simulink model "cardio"  (Simulink 7.2)
settings: Solver=ode45  StartTime=0.0  StopTime=10.0  RelTol=1e-3
undefined symbols (not defined in the file): ln
(part 1 of 2)
settings Model: Creator=hp  LastModifiedBy=hp

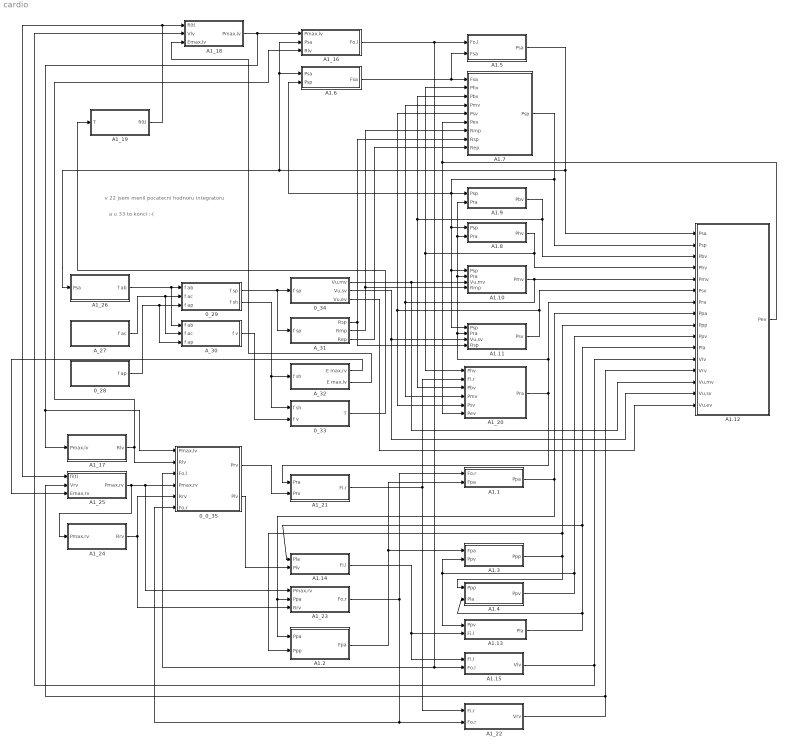
== system cardio ==
  note: v 22 jsem menil pocatecni hodnoru integratoru
  note: a u 33 to konci :-(
  0_0_35 : Subsystem
  0_28 : Subsystem
  0_29 : Subsystem
  0_33 : Subsystem
  0_34 : Subsystem
  A1.1 : Subsystem
  A1.10 : Subsystem
  A1.11 : Subsystem
  A1.12 : Subsystem
  A1.13 : Subsystem
  A1.14 : Subsystem
  A1.15 : Subsystem
  A1.2 : Subsystem
  A1.3 : Subsystem
  A1.4 : Subsystem
  A1.5 : Subsystem
  A1.6 : Subsystem
  A1.7 : Subsystem
  A1.8 : Subsystem
  A1.9 : Subsystem
  A1_16 : Subsystem
  A1_17 : Subsystem
  A1_18 : Subsystem
  A1_19 : Subsystem
  A1_20 : Subsystem
  A1_21 : Subsystem
  A1_22 : Subsystem
  A1_23 : Subsystem
  A1_24 : Subsystem
  A1_25 : Subsystem
  A1_26 : Subsystem
  A_27 : Subsystem
  A_30 : Subsystem
  A_31 : Subsystem
  A_32 : Subsystem
  wires:
  A1.10/1(Pmv) -> A1.12/5(Pmv), A1.7/4(Pmv), A1_20/4(Pmv)
  A1.11/1(Psv) -> A1.12/6(Psv), A1.7/5(Psv), A1_20/5(Psv)
  A1.3/1(Ppp) -> A1.4/1(Ppp), A1.12/9(Ppp), A1.2/2(Ppp)
  A1.15/1(Vlv) -> A1.12/12(Vlv), A1_18/2(Vlv)
  A1_26/1(f ab) -> 0_29/1(f ab), A_30/1(f ab)
  A_27/1(f ac) -> 0_29/2(f ac), A_30/2(f ac)
  0_28/1(f ap) -> 0_29/3(f ap), A_30/3(f ap)
  0_29/1(f sp) -> 0_34/1(f sp), A_31/1(f sp)
  0_29/2(f sh) -> A_32/1(f sh), 0_33/1(f sh)
  A1.4/1(Ppv) -> A1.12/10(Ppv), A1.3/2(Ppv), A1.13/1(Ppv)
  A1.13/1(Pla) -> A1.4/2(Pla), A1.12/11(Pla), A1.14/1(Pla)
  A1.8/1(Phv) -> A1.12/4(Phv), A1_20/1(Phv), A1.7/2(Phv)
  A1.9/1(Pbv) -> A1.12/3(Pbv), A1.7/3(Pbv), A1_20/3(Pbv)
  A1.7/1(Psp) -> A1.12/2(Psp), A1.9/1(Psp), A1.8/1(Psp), A1.10/1(Psp), A1.11/1(Psp), A1.6/2(Psp)
  A1.5/1(Psa) -> A1.12/1(Psa), A1.6/1(Psa), A1_16/2(Psa), A1_26/1(Psa)
  A1_20/1(Pra) -> A1.12/7(Pra), A1.10/2(Pra), A1.8/2(Pra), A1.9/2(Pra), A1.11/2(Pra), A1_21/1(Pra)
  A1.1/1(Ppa) -> A1.12/8(Ppa), A1.2/1(Ppa), A1_23/2(Ppa)
  A1_22/1(Vrv) -> A1.12/13(Vrv), A1_25/2(Vrv)
  A1_16/1(Fo,l) -> A1.5/1(Fo,l), A1.15/2(Fo,l), 0_0_35/3(Fo,l)
  A1.6/1(Fsa) -> A1.7/1(Fsa), A1.5/2(Fsa)
  A1.12/1(Pev) -> A1.7/6(Pev), A1_20/6(Pev)
  0_34/1(Vu,mv) -> A1.10/3(Vu,mv), A1.12/14(Vu,mv)
  0_34/2(Vu,sv) -> A1.11/3(Vu,sv), A1.12/15(Vu,sv)
  A1_21/1(Fi,r) -> A1_20/2(Fi,r), A1_22/1(Fi,r)
  A1.14/1(Fi,l) -> A1.15/1(Fi,l), A1.13/2(Fi,l)
  A1_23/1(Fo,r) -> A1.1/1(Fo,r), A1_22/2(Fo,r), 0_0_35/6(Fo,r)
  A1.2/1(Fpa) -> A1.3/1(Fpa), A1.1/2(Fpa)
  A1_18/1(Pmax,lv) -> A1_16/1(Pmax,lv), A1_17/1(Pmax,lv), 0_0_35/1(Pmax,lv)
  0_0_35/1(Prv) -> A1_21/2(Prv)
  0_0_35/2(Plv) -> A1.14/2(Plv)
  A1_25/1(Pmax,rv) -> A1_24/1(Pmax,rv), 0_0_35/4(Pmax,rv), A1_23/1(Pmax,rv)
  A1_24/1(Rrv) -> 0_0_35/5(Rrv), A1_23/3(Rrv)
  A1_17/1(Rlv) -> 0_0_35/2(Rlv), A1_16/3(Rlv)
  A1_19/1(fi(t)) -> A1_18/1(fi(t)), A1_25/1(fi(t))
  0_33/1(T) -> A1_19/1(T)
  A_31/1(Rsp) -> A1.7/8(Rsp), A1.11/4(Rsp)
  A_31/2(Rmp) -> A1.7/7(Rmp), A1.10/4(Rmp)
  A_31/3(Rep) -> A1.7/9(Rep)
  A_32/2(E max,lv) -> A1_18/3(Emax,lv)
  A_32/1(E max,rv) -> A1_25/3(Emax,rv)
  0_34/3(Vu,ev) -> A1.12/16(Vu,ev)
  A_30/1(f v) -> 0_33/2(f v)

== system cardio/0_0_35 ==
  Pmax,lv : Inport  OutDataType=fixdt(1, 16)  OutScaling=2^0
  Rlv : Inport  Port=2  OutDataType=fixdt(1, 16)  OutScaling=2^0
  Fo,l : Inport  Port=3  OutDataType=fixdt(1, 16)  OutScaling=2^0
  Pmax,rv : Inport  Port=4  OutDataType=fixdt(1, 16)  OutScaling=2^0
  Rrv : Inport  Port=5  OutDataType=fixdt(1, 16)  OutScaling=2^0
  Fo,r : Inport  Port=6  OutDataType=fixdt(1, 16)  OutScaling=2^0
  Add : Sum  Inputs=+-  OutDataType=fixdt(1, 16)  OutScaling=2^-10
  Add1 : Sum  Inputs=+-  OutDataType=fixdt(1, 16)  OutScaling=2^-10
  Product : Product  OutDataType=fixdt(1, 16)  OutScaling=2^0  RndMeth=Zero
  Product1 : Product  OutDataType=fixdt(1, 16)  OutScaling=2^0  RndMeth=Zero
  Prv : Outport  OutDataType=fixdt(1, 16)  OutScaling=2^0
  Plv : Outport  Port=2  OutDataType=fixdt(1, 16)  OutScaling=2^0
  wires:
  Product1/1 -> Add1/2
  Fo,r/1 -> Product1/2
  Rrv/1 -> Product1/1
  Pmax,rv/1 -> Add1/1
  Product/1 -> Add/2
  Fo,l/1 -> Product/2
  Rlv/1 -> Product/1
  Pmax,lv/1 -> Add/1
  Add/1 -> Plv/1
  Add1/1 -> Prv/1

== system cardio/0_28 ==
  1/tau p : Gain  Gain=1/2  ParameterDataType=sfix(16)  ParameterScaling=2^0  OutDataType=sfix(16)  OutScaling=2^0
  G ap : Constant  Value=23.29  OutDataType=sfix(16)  OutScaling=2^0
  Integrator : Integrator
  Subtract : Sum  Inputs=+-  OutDataType=sfix(16)  OutScaling=2^-10
  V T : Constant  Value=0.583  OutDataType=sfix(16)  OutScaling=2^0
  fi ap : Product  OutDataType=sfix(16)  OutScaling=2^0  RndMeth=Zero
  f ap : Outport  OutDataType=sfix(16)  OutScaling=2^0
  wires:
  V T/1 -> fi ap/2
  G ap/1 -> fi ap/1
  fi ap/1 -> Subtract/1
  Subtract/1 -> 1/tau p/1
  1/tau p/1 -> Integrator/1
  Integrator/1 -> Subtract/2, f ap/1

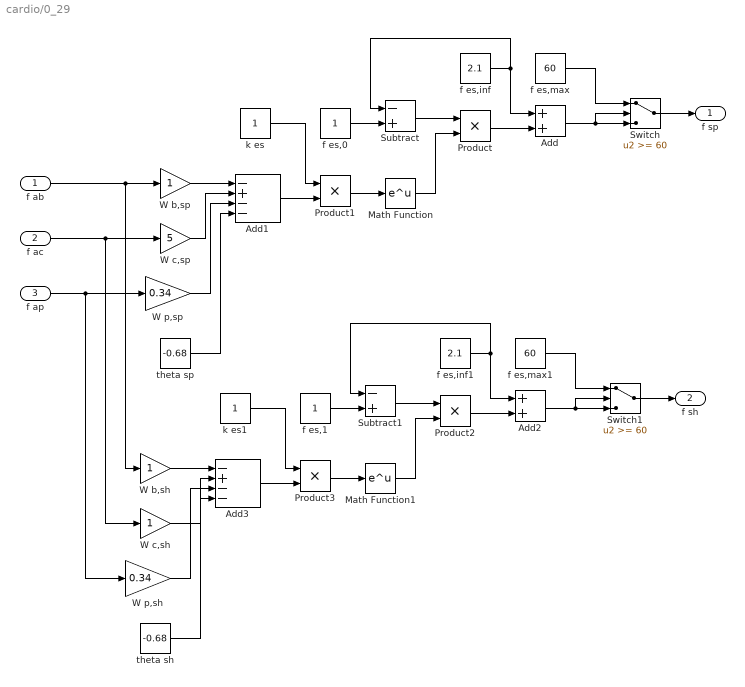
== system cardio/0_29 ==
  f ab : Inport  OutDataType=sfix(16)  OutScaling=2^0
  f ac : Inport  Port=2  OutDataType=sfix(16)  OutScaling=2^0
  f ap : Inport  Port=3  OutDataType=sfix(16)  OutScaling=2^0
  Add : Sum  OutDataType=sfix(16)  OutScaling=2^-10
  Add1 : Sum  Inputs=-+--  OutDataType=sfix(16)  OutScaling=2^-10
  Add2 : Sum  OutDataType=sfix(16)  OutScaling=2^-10
  Add3 : Sum  Inputs=-+--  OutDataType=sfix(16)  OutScaling=2^-10
  Math Function : Math  OutDataType=sfix(16)  OutScaling=2^0  SaturateOnIntegerOverflow=on
  Math Function1 : Math  OutDataType=sfix(16)  OutScaling=2^0  SaturateOnIntegerOverflow=on
  Product{,1..3} (4 alike) : Product  OutDataType=sfix(16)  OutScaling=2^0  RndMeth=Zero
  Subtract : Sum  Inputs=-+  OutDataType=sfix(16)  OutScaling=2^-10
  Subtract1 : Sum  Inputs=-+  OutDataType=sfix(16)  OutScaling=2^-10
  Switch : Switch  Threshold=60  OutDataType=sfix(16)  OutScaling=2^0
  Switch1 : Switch  Threshold=60  OutDataType=sfix(16)  OutScaling=2^0
  W b,sh : Gain  ParameterDataType=sfix(16)  ParameterScaling=2^0  OutDataType=sfix(16)  OutScaling=2^0
  W b,sp : Gain  ParameterDataType=sfix(16)  ParameterScaling=2^0  OutDataType=sfix(16)  OutScaling=2^0
  W c,sh : Gain  ParameterDataType=sfix(16)  ParameterScaling=2^0  OutDataType=sfix(16)  OutScaling=2^0
  W c,sp : Gain  Gain=5  ParameterDataType=sfix(16)  ParameterScaling=2^0  OutDataType=sfix(16)  OutScaling=2^0
  W p,sh : Gain  Gain=0.34  ParameterDataType=sfix(16)  ParameterScaling=2^0  OutDataType=sfix(16)  OutScaling=2^0
  W p,sp : Gain  Gain=0.34  ParameterDataType=sfix(16)  ParameterScaling=2^0  OutDataType=sfix(16)  OutScaling=2^0
  f es,0 : Constant  OutDataType=sfix(16)  OutScaling=2^0
  f es,1 : Constant  OutDataType=sfix(16)  OutScaling=2^0
  f es,inf : Constant  Value=2.1  OutDataType=sfix(16)  OutScaling=2^0
  f es,inf1 : Constant  Value=2.1  OutDataType=sfix(16)  OutScaling=2^0
  f es,max : Constant  Value=60  OutDataType=sfix(16)  OutScaling=2^0
  f es,max1 : Constant  Value=60  OutDataType=sfix(16)  OutScaling=2^0
  k es : Constant  OutDataType=sfix(16)  OutScaling=2^0
  k es1 : Constant  OutDataType=sfix(16)  OutScaling=2^0
  theta sh : Constant  Value=-0.68  OutDataType=sfix(16)  OutScaling=2^0
  theta sp : Constant  Value=-0.68  OutDataType=sfix(16)  OutScaling=2^0
  f sp : Outport  OutDataType=sfix(16)  OutScaling=2^0
  f sh : Outport  Port=2  OutDataType=sfix(16)  OutScaling=2^0
  wires:
  Add3/1 -> Product3/2
  theta sh/1 -> Add3/4
  W p,sh/1 -> Add3/3
  W c,sh/1 -> Add3/2
  W b,sh/1 -> Add3/1
  k es1/1 -> Product3/1
  Product3/1 -> Math Function1/1
  Math Function1/1 -> Product2/2
  f es,1/1 -> Subtract1/2
  Subtract1/1 -> Product2/1
  Product2/1 -> Add2/2
  f es,inf1/1 -> Subtract1/1, Add2/1
  Add2/1 -> Switch1/3, Switch1/2
  Switch1/1 -> f sh/1
  f es,max1/1 -> Switch1/1
  Add1/1 -> Product1/2
  theta sp/1 -> Add1/4
  W p,sp/1 -> Add1/3
  f ap/1 -> W p,sh/1, W p,sp/1
  f ac/1 -> W c,sh/1, W c,sp/1
  W c,sp/1 -> Add1/2
  f ab/1 -> W b,sh/1, W b,sp/1
  W b,sp/1 -> Add1/1
  k es/1 -> Product1/1
  Product1/1 -> Math Function/1
  Math Function/1 -> Product/2
  f es,0/1 -> Subtract/2
  Subtract/1 -> Product/1
  Product/1 -> Add/2
  f es,inf/1 -> Subtract/1, Add/1
  Add/1 -> Switch/3, Switch/2
  Switch/1 -> f sp/1
  f es,max/1 -> Switch/1

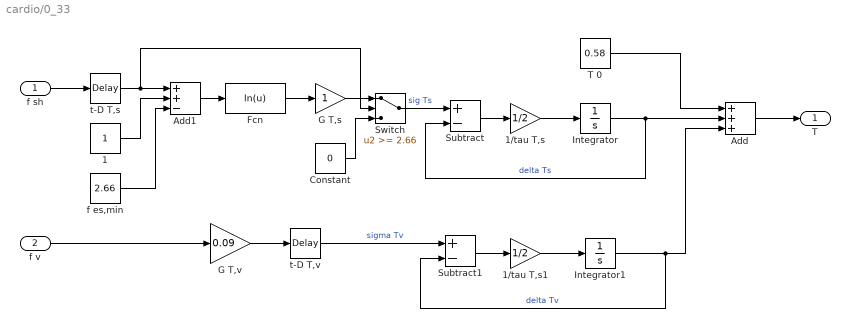
== system cardio/0_33 ==
  f sh : Inport  OutDataType=sfix(16)  OutScaling=2^0
  f v : Inport  Port=2  OutDataType=sfix(16)  OutScaling=2^0
  1 : Constant  OutDataType=sfix(16)  OutScaling=2^0
  1/tau T,s : Gain  Gain=1/2  ParameterDataType=sfix(16)  ParameterScaling=2^0  OutDataType=sfix(16)  OutScaling=2^0
  1/tau T,s1 : Gain  Gain=1/2  ParameterDataType=sfix(16)  ParameterScaling=2^0  OutDataType=sfix(16)  OutScaling=2^0
  Add : Sum  Inputs=+++  OutDataType=sfix(16)  OutScaling=2^-10
  Add1 : Sum  Inputs=++-  OutDataType=sfix(16)  OutScaling=2^-10
  Constant : Constant  Value=0  OutDataType=sfix(16)  OutScaling=2^0
  Fcn : Fcn  Expr=ln(u)
  G T,s : Gain  ParameterDataType=sfix(16)  ParameterScaling=2^0  OutDataType=sfix(16)  OutScaling=2^0
  G T,v : Gain  Gain=0.09  ParameterDataType=sfix(16)  ParameterScaling=2^0  OutDataType=sfix(16)  OutScaling=2^0
  Integrator : Integrator
  Integrator1 : Integrator
  Subtract : Sum  Inputs=+-  OutDataType=sfix(16)  OutScaling=2^-10
  Subtract1 : Sum  Inputs=+-  OutDataType=sfix(16)  OutScaling=2^-10
  Switch : Switch  Threshold=2.66  OutDataType=sfix(16)  OutScaling=2^0
  T 0 : Constant  Value=0.58  OutDataType=sfix(16)  OutScaling=2^0
  f es,min : Constant  Value=2.66  OutDataType=sfix(16)  OutScaling=2^0
  t-D T,s : TransportDelay  DelayTime=2
  t-D T,v : TransportDelay  DelayTime=0.2
  T : Outport  OutDataType=sfix(16)  OutScaling=2^0
  wires:
  Switch/1 -> Subtract/1  "sig Ts"
  Constant/1 -> Switch/3
  G T,s/1 -> Switch/1
  Add1/1 -> Fcn/1
  f es,min/1 -> Add1/3
  1/1 -> Add1/2
  t-D T,s/1 -> Add1/1, Switch/2
  f sh/1 -> t-D T,s/1
  Fcn/1 -> G T,s/1
  t-D T,v/1 -> Subtract1/1  "sigma Tv"
  G T,v/1 -> t-D T,v/1
  f v/1 -> G T,v/1
  T 0/1 -> Add/1
  Add/1 -> T/1
  Subtract1/1 -> 1/tau T,s1/1
  Integrator/1 -> Add/2, Subtract/2  "delta Ts"
  Subtract/1 -> 1/tau T,s/1
  1/tau T,s/1 -> Integrator/1
  1/tau T,s1/1 -> Integrator1/1
  Integrator1/1 -> Subtract1/2, Add/3  "delta Tv"

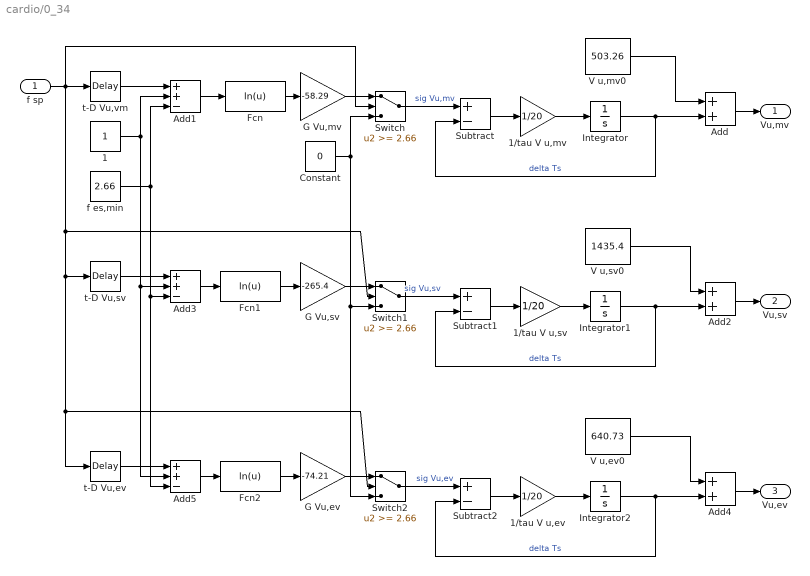
== system cardio/0_34 ==
  f sp : Inport  OutDataType=sfix(16)  OutScaling=2^0
  1 : Constant  OutDataType=sfix(16)  OutScaling=2^0
  1/tau V u,ev : Gain  Gain=1/20  ParameterDataType=sfix(16)  ParameterScaling=2^0  OutDataType=sfix(16)  OutScaling=2^0
  1/tau V u,mv : Gain  Gain=1/20  ParameterDataType=sfix(16)  ParameterScaling=2^0  OutDataType=sfix(16)  OutScaling=2^0
  1/tau V u,sv : Gain  Gain=1/20  ParameterDataType=sfix(16)  ParameterScaling=2^0  OutDataType=sfix(16)  OutScaling=2^0
  Add : Sum  OutDataType=sfix(16)  OutScaling=2^-10
  Add1 : Sum  Inputs=++-  OutDataType=sfix(16)  OutScaling=2^-10
  Add2 : Sum  OutDataType=sfix(16)  OutScaling=2^-10
  Add3 : Sum  Inputs=++-  OutDataType=sfix(16)  OutScaling=2^-10
  Add4 : Sum  OutDataType=sfix(16)  OutScaling=2^-10
  Add5 : Sum  Inputs=++-  OutDataType=sfix(16)  OutScaling=2^-10
  Constant : Constant  Value=0  OutDataType=sfix(16)  OutScaling=2^0
  Fcn : Fcn  Expr=ln(u)
  Fcn1 : Fcn  Expr=ln(u)
  Fcn2 : Fcn  Expr=ln(u)
  G Vu,ev : Gain  Gain=-74.21  ParameterDataType=sfix(16)  ParameterScaling=2^0  OutDataType=sfix(16)  OutScaling=2^0
  G Vu,mv : Gain  Gain=-58.29  ParameterDataType=sfix(16)  ParameterScaling=2^0  OutDataType=sfix(16)  OutScaling=2^0
  G Vu,sv : Gain  Gain=-265.4  ParameterDataType=sfix(16)  ParameterScaling=2^0  OutDataType=sfix(16)  OutScaling=2^0
  Integrator : Integrator
  Integrator1 : Integrator
  Integrator2 : Integrator
  Subtract : Sum  Inputs=+-  OutDataType=sfix(16)  OutScaling=2^-10
  Subtract1 : Sum  Inputs=+-  OutDataType=sfix(16)  OutScaling=2^-10
  Subtract2 : Sum  Inputs=+-  OutDataType=sfix(16)  OutScaling=2^-10
  Switch : Switch  Threshold=2.66  OutDataType=sfix(16)  OutScaling=2^0
  Switch1 : Switch  Threshold=2.66  OutDataType=sfix(16)  OutScaling=2^0
  Switch2 : Switch  Threshold=2.66  OutDataType=sfix(16)  OutScaling=2^0
  V u,ev0 : Constant  Value=640.73  OutDataType=sfix(16)  OutScaling=2^0
  V u,mv0 : Constant  Value=503.26  OutDataType=sfix(16)  OutScaling=2^0
  V u,sv0 : Constant  Value=1435.4  OutDataType=sfix(16)  OutScaling=2^0
  f es,min : Constant  Value=2.66  OutDataType=sfix(16)  OutScaling=2^0
  t-D Vu,ev : TransportDelay  DelayTime=2
  t-D Vu,sv : TransportDelay  DelayTime=2
  t-D Vu,vm : TransportDelay  DelayTime=2
  Vu,mv : Outport  OutDataType=sfix(16)  OutScaling=2^0
  Vu,sv : Outport  Port=2  OutDataType=sfix(16)  OutScaling=2^0
  Vu,ev : Outport  Port=3  OutDataType=sfix(16)  OutScaling=2^0
  wires:
  Add4/1 -> Vu,ev/1
  Switch2/1 -> Subtract2/1  "sig Vu,ev"
  G Vu,ev/1 -> Switch2/1
  Add5/1 -> Fcn2/1
  t-D Vu,ev/1 -> Add5/1
  Fcn2/1 -> G Vu,ev/1
  V u,ev0/1 -> Add4/1
  Integrator2/1 -> Add4/2, Subtract2/2  "delta Ts"
  Subtract2/1 -> 1/tau V u,ev/1
  1/tau V u,ev/1 -> Integrator2/1
  Add2/1 -> Vu,sv/1
  Switch1/1 -> Subtract1/1  "sig Vu,sv"
  G Vu,sv/1 -> Switch1/1
  Add3/1 -> Fcn1/1
  t-D Vu,sv/1 -> Add3/1
  Fcn1/1 -> G Vu,sv/1
  V u,sv0/1 -> Add2/1
  Integrator1/1 -> Add2/2, Subtract1/2  "delta Ts"
  Subtract1/1 -> 1/tau V u,sv/1
  1/tau V u,sv/1 -> Integrator1/1
  Add/1 -> Vu,mv/1
  Switch/1 -> Subtract/1  "sig Vu,mv"
  Constant/1 -> Switch2/3, Switch1/3, Switch/3
  G Vu,mv/1 -> Switch/1
  Add1/1 -> Fcn/1
  f es,min/1 -> Add5/3, Add3/3, Add1/3
  1/1 -> Add5/2, Add3/2, Add1/2
  t-D Vu,vm/1 -> Add1/1
  f sp/1 -> Switch1/2, Switch2/2, t-D Vu,ev/1, t-D Vu,sv/1, Switch/2, t-D Vu,vm/1
  Fcn/1 -> G Vu,mv/1
  V u,mv0/1 -> Add/1
  Integrator/1 -> Add/2, Subtract/2  "delta Ts"
  Subtract/1 -> 1/tau V u,mv/1
  1/tau V u,mv/1 -> Integrator/1

== system cardio/A1.1 ==
  Fo,r : Inport  OutDataType=sfix(16)  OutScaling=2^0
  Fpa : Inport  Port=2  OutDataType=sfix(16)  OutScaling=2^0
  Add : Sum  Inputs=+-  OutDataType=sfix(16)  OutScaling=2^-10
  Constant : Constant  OutDataType=sfix(16)  OutScaling=2^0
  Cpa : Constant  Value=0.76  OutDataType=sfix(16)  OutScaling=2^0
  Divide : Product  Inputs=*/  OutDataType=sfix(16)  OutScaling=2^-10
  Integrator : Integrator
  Product : Product  OutDataType=sfix(16)  OutScaling=2^0  RndMeth=Zero
  Ppa : Outport  OutDataType=sfix(16)  OutScaling=2^0
  wires:
  Fpa/1 -> Add/2
  Fo,r/1 -> Add/1
  Cpa/1 -> Divide/2
  Integrator/1 -> Ppa/1
  Product/1 -> Integrator/1
  Add/1 -> Product/2
  Divide/1 -> Product/1
  Constant/1 -> Divide/1

== system cardio/A1.10 ==
  note: Rm
  Psp : Inport  OutDataType=sfix(16)  OutScaling=2^0
  Pra : Inport  Port=2  OutDataType=sfix(16)  OutScaling=2^0
  Vu,mv : Inport  Port=3  OutDataType=sfix(16)  OutScaling=2^0
  Rmp : Inport  Port=4  OutDataType=sfix(16)  OutScaling=2^0
  Add : Sum  Inputs=+-  OutDataType=sfix(16)  OutScaling=2^-10
  Add1 : Sum  Inputs=-+  OutDataType=sfix(16)  OutScaling=2^-10
  Add2 : Sum  Inputs=+--  OutDataType=sfix(16)  OutScaling=2^-10
  Cmv : Constant  Value=15.71  OutDataType=sfix(16)  OutScaling=2^0
  Constant : Constant  OutDataType=sfix(16)  OutScaling=2^0
  Derivative : Derivative
  Divide : Product  Inputs=*/  OutDataType=sfix(16)  OutScaling=2^-10
  Divide1 : Product  Inputs=*/  OutDataType=sfix(16)  OutScaling=2^-10
  Divide2 : Product  Inputs=*/  OutDataType=sfix(16)  OutScaling=2^-10
  Integrator : Integrator
  Product : Product  OutDataType=sfix(16)  OutScaling=2^0  RndMeth=Zero
  Rmv : Constant  Value=0.05  OutDataType=sfix(16)  OutScaling=2^0
  Pmv : Outport  OutDataType=sfix(16)  OutScaling=2^0
  wires:
  Derivative/1 -> Add2/3
  Vu,mv/1 -> Derivative/1
  Add2/1 -> Product/2
  Divide2/1 -> Add2/2
  Divide1/1 -> Add2/1
  Rmv/1 -> Divide2/2
  Add1/1 -> Divide2/1
  Rmp/1 -> Divide1/2
  Add/1 -> Divide1/1
  Pra/1 -> Add1/1
  Psp/1 -> Add/1
  Integrator/1 -> Add1/2, Pmv/1, Add/2
  Product/1 -> Integrator/1
  Divide/1 -> Product/1
  Cmv/1 -> Divide/2
  Constant/1 -> Divide/1

== system cardio/A1.11 ==
  note: Rs
  Psp : Inport  OutDataType=sfix(16)  OutScaling=2^0
  Pra : Inport  Port=2  OutDataType=sfix(16)  OutScaling=2^0
  Vu,sv : Inport  Port=3  OutDataType=sfix(16)  OutScaling=2^0
  Rsp : Inport  Port=4  OutDataType=sfix(16)  OutScaling=2^0
  Add : Sum  Inputs=+-  OutDataType=sfix(16)  OutScaling=2^-10
  Add1 : Sum  Inputs=-+  OutDataType=sfix(16)  OutScaling=2^-10
  Add2 : Sum  Inputs=+--  OutDataType=sfix(16)  OutScaling=2^-10
  Constant : Constant  OutDataType=sfix(16)  OutScaling=2^0
  Csv : Constant  Value=61.11  OutDataType=sfix(16)  OutScaling=2^0
  Derivative : Derivative
  Divide : Product  Inputs=*/  OutDataType=sfix(16)  OutScaling=2^-10
  Divide1 : Product  Inputs=*/  OutDataType=sfix(16)  OutScaling=2^-10
  Divide2 : Product  Inputs=*/  OutDataType=sfix(16)  OutScaling=2^-10
  Integrator : Integrator
  Product : Product  OutDataType=sfix(16)  OutScaling=2^0  RndMeth=Zero
  Rsv : Constant  Value=0.038  OutDataType=sfix(16)  OutScaling=2^0
  Psv : Outport  OutDataType=sfix(16)  OutScaling=2^0
  wires:
  Derivative/1 -> Add2/3
  Vu,sv/1 -> Derivative/1
  Add2/1 -> Product/2
  Divide2/1 -> Add2/2
  Divide1/1 -> Add2/1
  Rsv/1 -> Divide2/2
  Add1/1 -> Divide2/1
  Rsp/1 -> Divide1/2
  Add/1 -> Divide1/1
  Pra/1 -> Add1/1
  Psp/1 -> Add/1
  Integrator/1 -> Add1/2, Psv/1, Add/2
  Product/1 -> Integrator/1
  Divide/1 -> Product/1
  Csv/1 -> Divide/2
  Constant/1 -> Divide/1

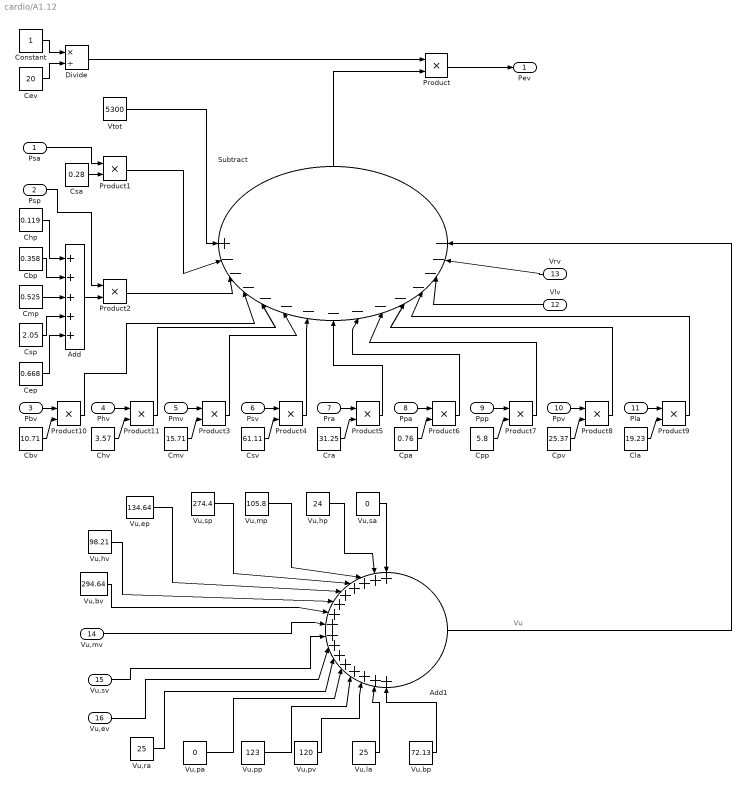
== system cardio/A1.12 ==
  note: Vu
  Psa : Inport  OutDataType=sfix(16)  OutScaling=2^0
  Psp : Inport  Port=2  OutDataType=sfix(16)  OutScaling=2^0
  Pbv : Inport  Port=3  OutDataType=sfix(16)  OutScaling=2^0
  Phv : Inport  Port=4  OutDataType=sfix(16)  OutScaling=2^0
  Pmv : Inport  Port=5  OutDataType=sfix(16)  OutScaling=2^0
  Psv : Inport  Port=6  OutDataType=sfix(16)  OutScaling=2^0
  Pra : Inport  Port=7  OutDataType=sfix(16)  OutScaling=2^0
  Ppa : Inport  Port=8  OutDataType=sfix(16)  OutScaling=2^0
  Ppp : Inport  Port=9  OutDataType=sfix(16)  OutScaling=2^0
  Ppv : Inport  Port=10  OutDataType=sfix(16)  OutScaling=2^0
  Pla : Inport  Port=11  OutDataType=sfix(16)  OutScaling=2^0
  Vlv : Inport  Orientation=left  Port=12  OutDataType=sfix(16)  OutScaling=2^0
  Vrv : Inport  Orientation=left  Port=13  OutDataType=sfix(16)  OutScaling=2^0
  Vu,mv : Inport  Port=14  OutDataType=sfix(16)  OutScaling=2^0
  Vu,sv : Inport  Port=15  OutDataType=sfix(16)  OutScaling=2^0
  Vu,ev : Inport  Port=16  OutDataType=sfix(16)  OutScaling=2^0
  Add : Sum  Inputs=+++++  OutDataType=sfix(16)  OutScaling=2^-10
  Add1 : Sum  Inputs=++++++++++++++++  OutDataType=sfix(16)  OutScaling=2^-10
  Cbp : Constant  Value=0.358  OutDataType=sfix(16)  OutScaling=2^0
  Cbv : Constant  Value=10.71  OutDataType=sfix(16)  OutScaling=2^0
  Cep : Constant  Value=0.668  OutDataType=sfix(16)  OutScaling=2^0
  Cev : Constant  Value=20  OutDataType=sfix(16)  OutScaling=2^0
  Chp : Constant  Value=0.119  OutDataType=sfix(16)  OutScaling=2^0
  Chv : Constant  Value=3.57  OutDataType=sfix(16)  OutScaling=2^0
  Cla : Constant  Value=19.23  OutDataType=sfix(16)  OutScaling=2^0
  Cmp : Constant  Value=0.525  OutDataType=sfix(16)  OutScaling=2^0
  Cmv : Constant  Value=15.71  OutDataType=sfix(16)  OutScaling=2^0
  Constant : Constant  OutDataType=sfix(16)  OutScaling=2^0
  Cpa : Constant  Value=0.76  OutDataType=sfix(16)  OutScaling=2^0
  Cpp : Constant  Value=5.8  OutDataType=sfix(16)  OutScaling=2^0
  Cpv : Constant  Value=25.37  OutDataType=sfix(16)  OutScaling=2^0
  Cra : Constant  Value=31.25  OutDataType=sfix(16)  OutScaling=2^0
  Csa : Constant  Value=0.28  OutDataType=sfix(16)  OutScaling=2^0
  Csp : Constant  Value=2.05  OutDataType=sfix(16)  OutScaling=2^0
  Csv : Constant  Value=61.11  OutDataType=sfix(16)  OutScaling=2^0
  Divide : Product  Inputs=*/  OutDataType=sfix(16)  OutScaling=2^-10
  Product{,1..11} (12 alike) : Product  OutDataType=sfix(16)  OutScaling=2^0  RndMeth=Zero
  Subtract : Sum  Orientation=up  Inputs=+--------------  OutDataType=sfix(16)  OutScaling=2^-10
  Vtot : Constant  Value=5300  OutDataType=sfix(16)  OutScaling=2^0
  Vu,bp : Constant  Value=72.13  OutDataType=sfix(16)  OutScaling=2^0
  Vu,bv : Constant  Value=294.64  OutDataType=sfix(16)  OutScaling=2^0
  Vu,ep : Constant  Value=134.64  OutDataType=sfix(16)  OutScaling=2^0
  Vu,hp : Constant  Value=24  OutDataType=sfix(16)  OutScaling=2^0
  Vu,hv : Constant  Value=98.21  OutDataType=sfix(16)  OutScaling=2^0
  Vu,la : Constant  Value=25  OutDataType=sfix(16)  OutScaling=2^0
  Vu,mp : Constant  Value=105.8  OutDataType=sfix(16)  OutScaling=2^0
  Vu,pa : Constant  Value=0  OutDataType=sfix(16)  OutScaling=2^0
  Vu,pp : Constant  Value=123  OutDataType=sfix(16)  OutScaling=2^0
  Vu,pv : Constant  Value=120  OutDataType=sfix(16)  OutScaling=2^0
  Vu,ra : Constant  Value=25  OutDataType=sfix(16)  OutScaling=2^0
  Vu,sa : Constant  Value=0  OutDataType=sfix(16)  OutScaling=2^0
  Vu,sp : Constant  Value=274.4  OutDataType=sfix(16)  OutScaling=2^0
  Pev : Outport  OutDataType=sfix(16)  OutScaling=2^0
  wires:
  Add1/1 -> Subtract/15
  Vu,sa/1 -> Add1/1
  Vu,hp/1 -> Add1/2
  Vu,mp/1 -> Add1/3
  Vu,sp/1 -> Add1/4
  Vu,ep/1 -> Add1/5
  Vu,hv/1 -> Add1/6
  Vu,bv/1 -> Add1/7
  Vu,mv/1 -> Add1/8
  Vu,sv/1 -> Add1/9
  Vu,ev/1 -> Add1/10
  Vu,ra/1 -> Add1/11
  Vu,pa/1 -> Add1/12
  Vu,pp/1 -> Add1/13
  Vu,pv/1 -> Add1/14
  Vu,la/1 -> Add1/15
  Vu,bp/1 -> Add1/16
  Subtract/1 -> Product/2
  Vrv/1 -> Subtract/14
  Vlv/1 -> Subtract/13
  Product3/1 -> Subtract/6
  Product2/1 -> Subtract/3
  Product1/1 -> Subtract/2
  Vtot/1 -> Subtract/1
  Product10/1 -> Subtract/4
  Product11/1 -> Subtract/5
  Chv/1 -> Product11/2
  Phv/1 -> Product11/1
  Cbv/1 -> Product10/2
  Pbv/1 -> Product10/1
  Product9/1 -> Subtract/12
  Product8/1 -> Subtract/11
  Product7/1 -> Subtract/10
  Product6/1 -> Subtract/9
  Product5/1 -> Subtract/8
  Product4/1 -> Subtract/7
  Cla/1 -> Product9/2
  Pla/1 -> Product9/1
  Cpv/1 -> Product8/2
  Ppv/1 -> Product8/1
  Cpp/1 -> Product7/2
  Ppp/1 -> Product7/1
  Cpa/1 -> Product6/2
  Ppa/1 -> Product6/1
  Cra/1 -> Product5/2
  Pra/1 -> Product5/1
  Csv/1 -> Product4/2
  Psv/1 -> Product4/1
  Cmv/1 -> Product3/2
  Pmv/1 -> Product3/1
  Psp/1 -> Product2/1
  Add/1 -> Product2/2
  Psa/1 -> Product1/1
  Csa/1 -> Product1/2
  Cep/1 -> Add/5
  Csp/1 -> Add/4
  Cmp/1 -> Add/3
  Cbp/1 -> Add/2
  Chp/1 -> Add/1
  Product/1 -> Pev/1
  Divide/1 -> Product/1
  Cev/1 -> Divide/2
  Constant/1 -> Divide/1

== system cardio/A1.13 ==
  Ppv : Inport  OutDataType=sfix(16)  OutScaling=2^0
  Fi,l : Inport  Port=2  OutDataType=sfix(16)  OutScaling=2^0
  Add : Sum  Inputs=+-  OutDataType=sfix(16)  OutScaling=2^-10
  Cla : Constant  Value=19.23  OutDataType=sfix(16)  OutScaling=2^0
  Constant : Constant  OutDataType=sfix(16)  OutScaling=2^0
  Divide : Product  Inputs=*/  OutDataType=sfix(16)  OutScaling=2^-10
  Divide1 : Product  Inputs=*/  OutDataType=sfix(16)  OutScaling=2^-10
  Integrator : Integrator
  Product : Product  OutDataType=sfix(16)  OutScaling=2^0  RndMeth=Zero
  Rpv : Constant  Value=0.0056  OutDataType=sfix(16)  OutScaling=2^0
  Subtract : Sum  Inputs=+-  OutDataType=sfix(16)  OutScaling=2^-10
  Pla : Outport  OutDataType=sfix(16)  OutScaling=2^0
  wires:
  Add/1 -> Product/2
  Fi,l/1 -> Add/2
  Divide1/1 -> Add/1
  Rpv/1 -> Divide1/2
  Subtract/1 -> Divide1/1
  Ppv/1 -> Subtract/1
  Divide/1 -> Product/1
  Product/1 -> Integrator/1
  Cla/1 -> Divide/2
  Constant/1 -> Divide/1
  Integrator/1 -> Subtract/2, Pla/1

== system cardio/A1.14 ==
  Pla : Inport  OutDataType=sfix(16)  OutScaling=2^0
  Plv : Inport  Port=2  OutDataType=sfix(16)  OutScaling=2^0
  Constant : Constant  Value=0  OutDataType=sfix(16)  OutScaling=2^0
  Divide : Product  Inputs=*/  OutDataType=sfix(16)  OutScaling=2^-10
  Rla : Constant  Value=0.0025  OutDataType=sfix(16)  OutScaling=2^0
  Subtract : Sum  Inputs=+-  OutDataType=sfix(16)  OutScaling=2^-10
  Switch : Switch  OutDataType=sfix(16)  OutScaling=2^0
  Fi,l : Outport  OutDataType=sfix(16)  OutScaling=2^0
  wires:
  Divide/1 -> Switch/3
  Switch/1 -> Fi,l/1
  Subtract/1 -> Switch/2, Divide/1
  Pla/1 -> Subtract/2
  Rla/1 -> Divide/2
  Constant/1 -> Switch/1
  Plv/1 -> Subtract/1

== system cardio/A1.15 ==
  Fi,l : Inport  OutDataType=sfix(16)  OutScaling=2^0
  Fo,l : Inport  Port=2  OutDataType=sfix(16)  OutScaling=2^0
  Integrator : Integrator
  Subtract : Sum  Inputs=+-  OutDataType=sfix(16)  OutScaling=2^-10
  Vlv : Outport  OutDataType=sfix(16)  OutScaling=2^0
  wires:
  Integrator/1 -> Vlv/1
  Subtract/1 -> Integrator/1
  Fo,l/1 -> Subtract/2
  Fi,l/1 -> Subtract/1

== system cardio/A1.2 ==
  Ppa : Inport  OutDataType=sfix(16)  OutScaling=2^0
  Ppp : Inport  Port=2  OutDataType=sfix(16)  OutScaling=2^0
  Add : Sum  Inputs=+--  OutDataType=sfix(16)  OutScaling=2^-10
  Constant : Constant  OutDataType=sfix(16)  OutScaling=2^0
  Divide : Product  Inputs=*/  OutDataType=sfix(16)  OutScaling=2^-10
  Integrator : Integrator
  Lpa : Constant  Value=0.00018  OutDataType=sfix(16)  OutScaling=2^0
  Product : Product  OutDataType=sfix(16)  OutScaling=2^0  RndMeth=Zero
  Product1 : Product  OutDataType=sfix(16)  OutScaling=2^0  RndMeth=Zero
  Rpa : Constant  Value=0.023  OutDataType=sfix(16)  OutScaling=2^0
  Fpa : Outport  OutDataType=sfix(16)  OutScaling=2^0
  wires:
  Integrator/1 -> Product1/2, Fpa/1
  Product/1 -> Integrator/1
  Add/1 -> Product/2
  Divide/1 -> Product/1
  Product1/1 -> Add/3
  Ppp/1 -> Add/2
  Ppa/1 -> Add/1
  Rpa/1 -> Product1/1
  Lpa/1 -> Divide/2
  Constant/1 -> Divide/1

== system cardio/A1.3 ==
  Fpa : Inport  OutDataType=sfix(16)  OutScaling=2^0
  Ppv : Inport  Port=2  OutDataType=sfix(16)  OutScaling=2^0
  Add : Sum  Inputs=-+  OutDataType=sfix(16)  OutScaling=2^-10
  Add1 : Sum  Inputs=+-  OutDataType=sfix(16)  OutScaling=2^-10
  Constant : Constant  OutDataType=sfix(16)  OutScaling=2^0
  Cpp : Constant  Value=5.8  OutDataType=sfix(16)  OutScaling=2^0
  Divide : Product  Inputs=*/  OutDataType=sfix(16)  OutScaling=2^-10
  Divide1 : Product  Inputs=*/  OutDataType=sfix(16)  OutScaling=2^-10
  Integrator : Integrator
  Product : Product  OutDataType=sfix(16)  OutScaling=2^0  RndMeth=Zero
  Rpp : Constant  Value=0.0894  OutDataType=sfix(16)  OutScaling=2^0
  Ppp : Outport  OutDataType=sfix(16)  OutScaling=2^0
  wires:
  Product/1 -> Integrator/1
  Add1/1 -> Product/2
  Divide/1 -> Product/1
  Divide1/1 -> Add1/2
  Fpa/1 -> Add1/1
  Rpp/1 -> Divide1/2
  Add/1 -> Divide1/1
  Integrator/1 -> Add/2, Ppp/1
  Ppv/1 -> Add/1
  Cpp/1 -> Divide/2
  Constant/1 -> Divide/1

== system cardio/A1.4 ==
  Ppp : Inport  OutDataType=sfix(16)  OutScaling=2^0
  Pla : Inport  Port=2  OutDataType=sfix(16)  OutScaling=2^0
  Add : Sum  Inputs=+-  OutDataType=sfix(16)  OutScaling=2^-10
  Add1 : Sum  Inputs=-+  OutDataType=sfix(16)  OutScaling=2^-10
  Add2 : Sum  Inputs=+-  OutDataType=sfix(16)  OutScaling=2^-10
  Constant : Constant  OutDataType=sfix(16)  OutScaling=2^0
  Cpv : Constant  Value=25.37  OutDataType=sfix(16)  OutScaling=2^0
  Divide : Product  Inputs=*/  OutDataType=sfix(16)  OutScaling=2^-10
  Divide1 : Product  Inputs=*/  OutDataType=sfix(16)  OutScaling=2^-10
  Divide2 : Product  Inputs=*/  OutDataType=sfix(16)  OutScaling=2^-10
  Integrator : Integrator
  Product : Product  OutDataType=sfix(16)  OutScaling=2^0  RndMeth=Zero
  Rpp : Constant  Value=0.0894  OutDataType=sfix(16)  OutScaling=2^0
  Rpv : Constant  Value=0.0056  OutDataType=sfix(16)  OutScaling=2^0
  Ppv : Outport  OutDataType=sfix(16)  OutScaling=2^0
  wires:
  Add2/1 -> Product/2
  Divide2/1 -> Add2/2
  Divide1/1 -> Add2/1
  Rpv/1 -> Divide2/2
  Rpp/1 -> Divide1/2
  Add/1 -> Divide1/1
  Add1/1 -> Divide2/1
  Pla/1 -> Add1/1
  Ppp/1 -> Add/1
  Integrator/1 -> Add1/2, Ppv/1, Add/2
  Product/1 -> Integrator/1
  Divide/1 -> Product/1
  Cpv/1 -> Divide/2
  Constant/1 -> Divide/1

== system cardio/A1.5 ==
  Fo,l : Inport  OutDataType=sfix(16)  OutScaling=2^0
  Fsa : Inport  Port=2  OutDataType=sfix(16)  OutScaling=2^0
  Constant : Constant  OutDataType=sfix(16)  OutScaling=2^0
  Csa : Constant  Value=0.28  OutDataType=sfix(16)  OutScaling=2^0
  Divide : Product  Inputs=*/  OutDataType=sfix(16)  OutScaling=2^-10
  Integrator : Integrator
  Product : Product  OutDataType=sfix(16)  OutScaling=2^0  RndMeth=Zero
  Subtract : Sum  Inputs=+-  OutDataType=sfix(16)  OutScaling=2^-10
  Psa : Outport  OutDataType=sfix(16)  OutScaling=2^0
  wires:
  Constant/1 -> Divide/1
  Csa/1 -> Divide/2
  Integrator/1 -> Psa/1
  Product/1 -> Integrator/1
  Fsa/1 -> Subtract/2
  Fo,l/1 -> Subtract/1
  Subtract/1 -> Product/1
  Divide/1 -> Product/2

== system cardio/A1.6 ==
  Psa : Inport  OutDataType=sfix(16)  OutScaling=2^0
  Psp : Inport  Port=2  OutDataType=sfix(16)  OutScaling=2^0
  Add : Sum  Inputs=+--  OutDataType=sfix(16)  OutScaling=2^-10
  Constant : Constant  OutDataType=sfix(16)  OutScaling=2^0
  Divide : Product  Inputs=*/  OutDataType=sfix(16)  OutScaling=2^-10
  Integrator : Integrator
  Lsa : Constant  Value=0.00022  OutDataType=sfix(16)  OutScaling=2^0
  Product : Product  OutDataType=sfix(16)  OutScaling=2^0  RndMeth=Zero
  Product1 : Product  OutDataType=sfix(16)  OutScaling=2^0  RndMeth=Zero
  Rsa : Constant  Value=0.06  OutDataType=sfix(16)  OutScaling=2^0
  Fsa : Outport  OutDataType=sfix(16)  OutScaling=2^0
  wires:
  Add/1 -> Product/2
  Product1/1 -> Add/3
  Psp/1 -> Add/2
  Psa/1 -> Add/1
  Rsa/1 -> Product1/1
  Integrator/1 -> Product1/2, Fsa/1
  Product/1 -> Integrator/1
  Divide/1 -> Product/1
  Lsa/1 -> Divide/2
  Constant/1 -> Divide/1

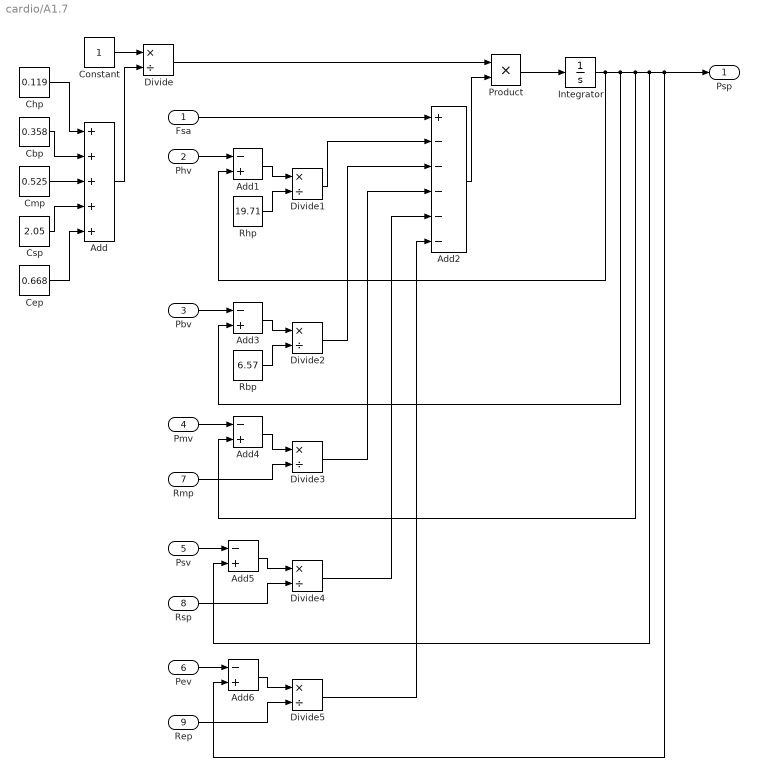
== system cardio/A1.7 ==
  Fsa : Inport  OutDataType=sfix(16)  OutScaling=2^0
  Phv : Inport  Port=2  OutDataType=sfix(16)  OutScaling=2^0
  Pbv : Inport  Port=3  OutDataType=sfix(16)  OutScaling=2^0
  Pmv : Inport  Port=4  OutDataType=sfix(16)  OutScaling=2^0
  Psv : Inport  Port=5  OutDataType=sfix(16)  OutScaling=2^0
  Pev : Inport  Port=6  OutDataType=sfix(16)  OutScaling=2^0
  Rmp : Inport  Port=7  OutDataType=sfix(16)  OutScaling=2^0
  Rsp : Inport  Port=8  OutDataType=sfix(16)  OutScaling=2^0
  Rep : Inport  Port=9  OutDataType=sfix(16)  OutScaling=2^0
  Add : Sum  Inputs=+++++  OutDataType=sfix(16)  OutScaling=2^-10
  Add{1,3..6} (5 alike) : Sum  Inputs=-+  OutDataType=sfix(16)  OutScaling=2^-10
  Add2 : Sum  Inputs=+-----  OutDataType=sfix(16)  OutScaling=2^-10
  Cbp : Constant  Value=0.358  OutDataType=sfix(16)  OutScaling=2^0
  Cep : Constant  Value=0.668  OutDataType=sfix(16)  OutScaling=2^0
  Chp : Constant  Value=0.119  OutDataType=sfix(16)  OutScaling=2^0
  Cmp : Constant  Value=0.525  OutDataType=sfix(16)  OutScaling=2^0
  Constant : Constant  OutDataType=sfix(16)  OutScaling=2^0
  Csp : Constant  Value=2.05  OutDataType=sfix(16)  OutScaling=2^0
  Divide{,1..5} (6 alike) : Product  Inputs=*/  OutDataType=sfix(16)  OutScaling=2^-10
  Integrator : Integrator
  Product : Product  OutDataType=sfix(16)  OutScaling=2^0  RndMeth=Zero
  Rbp : Constant  Value=6.57  OutDataType=sfix(16)  OutScaling=2^0
  Rhp : Constant  Value=19.71  OutDataType=sfix(16)  OutScaling=2^0
  Psp : Outport  OutDataType=sfix(16)  OutScaling=2^0
  wires:
  Divide5/1 -> Add2/6
  Rep/1 -> Divide5/2
  Add6/1 -> Divide5/1
  Pev/1 -> Add6/1
  Divide4/1 -> Add2/5
  Rsp/1 -> Divide4/2
  Add5/1 -> Divide4/1
  Psv/1 -> Add5/1
  Divide3/1 -> Add2/4
  Rmp/1 -> Divide3/2
  Add4/1 -> Divide3/1
  Pmv/1 -> Add4/1
  Divide2/1 -> Add2/3
  Rbp/1 -> Divide2/2
  Add3/1 -> Divide2/1
  Pbv/1 -> Add3/1
  Divide1/1 -> Add2/2
  Fsa/1 -> Add2/1
  Add2/1 -> Product/2
  Rhp/1 -> Divide1/2
  Add1/1 -> Divide1/1
  Phv/1 -> Add1/1
  Divide/1 -> Product/1
  Add/1 -> Divide/2
  Constant/1 -> Divide/1
  Cep/1 -> Add/5
  Csp/1 -> Add/4
  Chp/1 -> Add/1
  Cbp/1 -> Add/2
  Cmp/1 -> Add/3
  Product/1 -> Integrator/1
  Integrator/1 -> Add6/2, Psp/1, Add5/2, Add4/2, Add3/2, Add1/2

== system cardio/A1.8 ==
  Psp : Inport  OutDataType=sfix(16)  OutScaling=2^0
  Pra : Inport  Port=2  OutDataType=sfix(16)  OutScaling=2^0
  Add : Sum  Inputs=+-  OutDataType=sfix(16)  OutScaling=2^-10
  Add1 : Sum  Inputs=-+  OutDataType=sfix(16)  OutScaling=2^-10
  Add2 : Sum  Inputs=+-  OutDataType=sfix(16)  OutScaling=2^-10
  Chv : Constant  Value=3.57  OutDataType=sfix(16)  OutScaling=2^0
  Constant : Constant  OutDataType=sfix(16)  OutScaling=2^0
  Divide : Product  Inputs=*/  OutDataType=sfix(16)  OutScaling=2^-10
  Divide1 : Product  Inputs=*/  OutDataType=sfix(16)  OutScaling=2^-10
  Divide2 : Product  Inputs=*/  OutDataType=sfix(16)  OutScaling=2^-10
  Integrator : Integrator
  Product : Product  OutDataType=sfix(16)  OutScaling=2^0  RndMeth=Zero
  Rhp : Constant  Value=19.71  OutDataType=sfix(16)  OutScaling=2^0
  Rhv : Constant  Value=0.224  OutDataType=sfix(16)  OutScaling=2^0
  Phv : Outport  OutDataType=sfix(16)  OutScaling=2^0
  wires:
  Add2/1 -> Product/2
  Divide2/1 -> Add2/2
  Divide1/1 -> Add2/1
  Rhv/1 -> Divide2/2
  Add1/1 -> Divide2/1
  Rhp/1 -> Divide1/2
  Add/1 -> Divide1/1
  Pra/1 -> Add1/1
  Psp/1 -> Add/1
  Integrator/1 -> Add1/2, Phv/1, Add/2
  Product/1 -> Integrator/1
  Divide/1 -> Product/1
  Chv/1 -> Divide/2
  Constant/1 -> Divide/1

== system cardio/A1.9 ==
  note: Rbp
  Psp : Inport  OutDataType=sfix(16)  OutScaling=2^0
  Pra : Inport  Port=2  OutDataType=sfix(16)  OutScaling=2^0
  Add : Sum  Inputs=+-  OutDataType=sfix(16)  OutScaling=2^-10
  Add1 : Sum  Inputs=-+  OutDataType=sfix(16)  OutScaling=2^-10
  Add2 : Sum  Inputs=+-  OutDataType=sfix(16)  OutScaling=2^-10
  Cbv : Constant  Value=10.71  OutDataType=sfix(16)  OutScaling=2^0
  Constant : Constant  OutDataType=sfix(16)  OutScaling=2^0
  Divide : Product  Inputs=*/  OutDataType=sfix(16)  OutScaling=2^-10
  Divide1 : Product  Inputs=*/  OutDataType=sfix(16)  OutScaling=2^-10
  Divide2 : Product  Inputs=*/  OutDataType=sfix(16)  OutScaling=2^-10
  Integrator : Integrator
  Product : Product  OutDataType=sfix(16)  OutScaling=2^0  RndMeth=Zero
  Rbv : Constant  Value=0.075  OutDataType=sfix(16)  OutScaling=2^0
  Rhp : Constant  Value=6.57  OutDataType=sfix(16)  OutScaling=2^0
  Pbv : Outport  OutDataType=sfix(16)  OutScaling=2^0
  wires:
  Add2/1 -> Product/2
  Divide2/1 -> Add2/2
  Divide1/1 -> Add2/1
  Rbv/1 -> Divide2/2
  Add1/1 -> Divide2/1
  Rhp/1 -> Divide1/2
  Add/1 -> Divide1/1
  Pra/1 -> Add1/1
  Psp/1 -> Add/1
  Integrator/1 -> Add1/2, Pbv/1, Add/2
  Product/1 -> Integrator/1
  Divide/1 -> Product/1
  Cbv/1 -> Divide/2
  Constant/1 -> Divide/1

== system cardio/A1_16 ==
  Pmax,lv : Inport  OutDataType=sfix(16)  OutScaling=2^0
  Psa : Inport  Port=2  OutDataType=sfix(16)  OutScaling=2^0
  Rlv : Inport  Port=3  OutDataType=sfix(16)  OutScaling=2^0
  Constant : Constant  Value=0  OutDataType=sfix(16)  OutScaling=2^0
  Divide : Product  Inputs=*/  OutDataType=sfix(16)  OutScaling=2^-10
  Subtract : Sum  Inputs=+-  OutDataType=sfix(16)  OutScaling=2^-10
  Switch : Switch  OutDataType=sfix(16)  OutScaling=2^0
  Fo,l : Outport  OutDataType=sfix(16)  OutScaling=2^0
  wires:
  Switch/1 -> Fo,l/1
  Divide/1 -> Switch/3
  Rlv/1 -> Divide/2
  Subtract/1 -> Divide/1, Switch/2
  Constant/1 -> Switch/1
  Psa/1 -> Subtract/2
  Pmax,lv/1 -> Subtract/1

== system cardio/A1_17 ==
  Pmax,lv : Inport  OutDataType=fixdt(1, 16)  OutScaling=2^0
  Product : Product  OutDataType=fixdt(1, 16)  OutScaling=2^0  RndMeth=Zero
  kR,lv : Constant  Value=0.000375  OutDataType=fixdt(1, 16)  OutScaling=2^0
  Rlv : Outport  OutDataType=fixdt(1, 16)  OutScaling=2^0
  wires:
  kR,lv/1 -> Product/2
  Pmax,lv/1 -> Product/1
  Product/1 -> Rlv/1

== system cardio/A1_18 ==
  fi(t) : Inport  OutDataType=fixdt(1, 16)  OutScaling=2^0
  Vlv : Inport  Port=2  OutDataType=fixdt(1, 16)  OutScaling=2^0
  Emax,lv : Inport  Port=3  OutDataType=fixdt(1, 16)  OutScaling=2^0
  Add : Sum  OutDataType=fixdt(1, 16)  OutScaling=2^-10
  Add1 : Sum  Inputs=+-  OutDataType=fixdt(1, 16)  OutScaling=2^-10
  Constant : Constant  OutDataType=fixdt(1, 16)  OutScaling=2^0
  Constant1 : Constant  OutDataType=fixdt(1, 16)  OutScaling=2^0
  Math Function : Math  OutDataType=fixdt(1, 16)  OutScaling=2^0  SaturateOnIntegerOverflow=on
  Po,lv : Constant  Value=1.5  OutDataType=fixdt(1, 16)  OutScaling=2^0
  Product : Product  Inputs=3  OutDataType=fixdt(1, 16)  OutScaling=2^0  RndMeth=Zero
  Product1 : Product  Inputs=3  OutDataType=fixdt(1, 16)  OutScaling=2^0  RndMeth=Zero
  Product2 : Product  OutDataType=fixdt(1, 16)  OutScaling=2^0  RndMeth=Zero
  Subtract : Sum  Inputs=+-  OutDataType=fixdt(1, 16)  OutScaling=2^-10
  Subtract1 : Sum  Inputs=+-  OutDataType=fixdt(1, 16)  OutScaling=2^-10
  Vu,lv : Constant  Value=16.77  OutDataType=fixdt(1, 16)  OutScaling=2^0
  kE,lv : Constant  Value=0.014  OutDataType=fixdt(1, 16)  OutScaling=2^0
  Pmax,lv : Outport  OutDataType=fixdt(1, 16)  OutScaling=2^0
  wires:
  Math Function/1 -> Add1/1
  Product2/1 -> Math Function/1
  kE,lv/1 -> Product2/2
  Constant1/1 -> Add1/2
  Add1/1 -> Product1/3
  Po,lv/1 -> Product1/2
  Constant/1 -> Subtract1/1
  Subtract1/1 -> Product1/1
  Product1/1 -> Add/2
  Product/1 -> Add/1
  Add/1 -> Pmax,lv/1
  Subtract/1 -> Product/3
  Vu,lv/1 -> Subtract/2
  Vlv/1 -> Product2/1, Subtract/1
  Emax,lv/1 -> Product/2
  fi(t)/1 -> Subtract1/2, Product/1

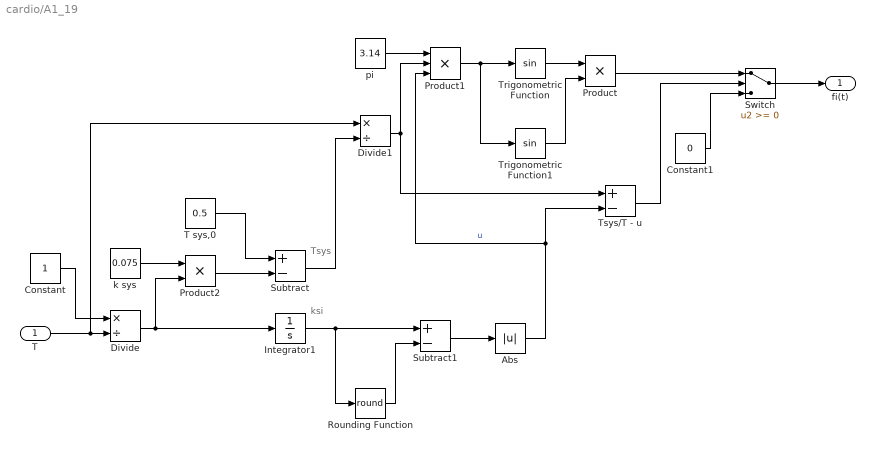
== system cardio/A1_19 ==
  note: Tsys
  note: ksi
  T : Inport  OutDataType=fixdt(1, 16)  OutScaling=2^0
  Abs : Abs  OutDataType=sfix(16)  OutScaling=2^0
  Constant : Constant  OutDataType=sfix(16)  OutScaling=2^0
  Constant1 : Constant  Value=0  OutDataType=sfix(16)  OutScaling=2^0
  Divide : Product  Inputs=*/  OutDataType=sfix(16)  OutScaling=2^-10
  Divide1 : Product  Inputs=*/  OutDataType=sfix(16)  OutScaling=2^-10
  Integrator1 : Integrator
  Product : Product  OutDataType=fixdt(1, 16)  OutScaling=2^0  RndMeth=Zero
  Product1 : Product  Inputs=3  OutDataType=fixdt(1, 16)  OutScaling=2^0  RndMeth=Zero
  Product2 : Product  OutDataType=sfix(16)  OutScaling=2^0  RndMeth=Zero
  Rounding Function : Rounding  Operator=round
  Subtract : Sum  Inputs=+-  OutDataType=sfix(16)  OutScaling=2^-10
  Subtract1 : Sum  Inputs=+-  OutDataType=sfix(16)  OutScaling=2^-10
  Switch : Switch  OutDataType=sfix(16)  OutScaling=2^0
  T sys,0 : Constant  Value=0.5  OutDataType=sfix(16)  OutScaling=2^0
  Trigonometric Function : Trigonometry
  Trigonometric Function1 : Trigonometry
  Tsys/T - u : Sum  Inputs=+-  OutDataType=sfix(16)  OutScaling=2^-10
  k sys : Constant  Value=0.075  OutDataType=sfix(16)  OutScaling=2^0
  pi : Constant  Value=3.14  OutDataType=fixdt(1, 16)  OutScaling=2^0
  fi(t) : Outport  OutDataType=fixdt(1, 16)  OutScaling=2^0
  wires:
  Divide1/1 -> Product1/2, Tsys/T - u/1
  pi/1 -> Product1/1
  Trigonometric Function1/1 -> Product/2
  Trigonometric Function/1 -> Product/1
  T sys,0/1 -> Subtract/1
  Product2/1 -> Subtract/2
  k sys/1 -> Product2/1
  Divide/1 -> Product2/2, Integrator1/1
  Constant/1 -> Divide/1
  T/1 -> Divide/2, Divide1/1
  Subtract/1 -> Divide1/2
  Integrator1/1 -> Subtract1/1, Rounding Function/1
  Product1/1 -> Trigonometric Function/1, Trigonometric Function1/1
  Rounding Function/1 -> Subtract1/2
  Subtract1/1 -> Abs/1
  Abs/1 -> Product1/3, Tsys/T - u/2  "u"
  Tsys/T - u/1 -> Switch/2
  Product/1 -> Switch/1
  Constant1/1 -> Switch/3
  Switch/1 -> fi(t)/1

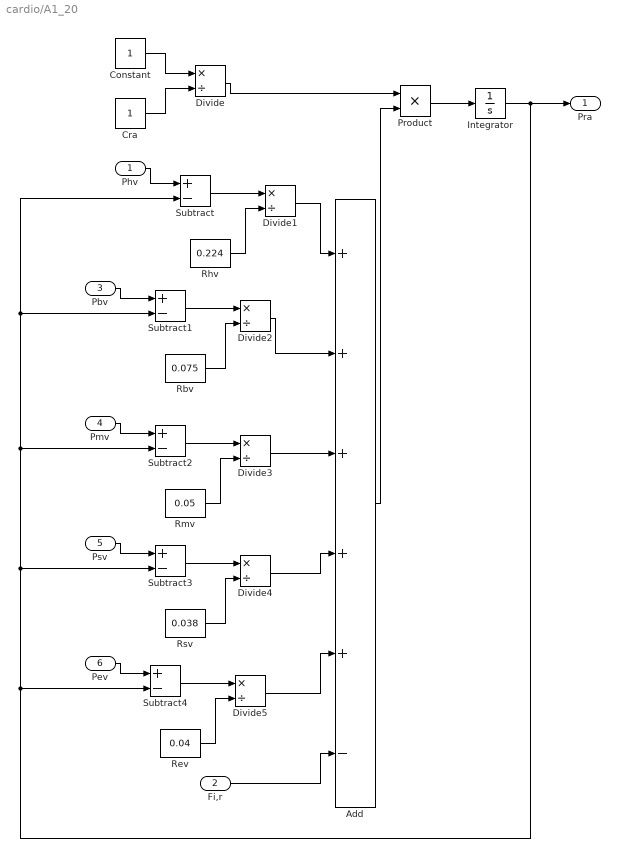
== system cardio/A1_20 ==
  Phv : Inport  OutDataType=sfix(16)  OutScaling=2^0
  Fi,r : Inport  Port=2  OutDataType=sfix(16)  OutScaling=2^0
  Pbv : Inport  Port=3  OutDataType=sfix(16)  OutScaling=2^0
  Pmv : Inport  Port=4  OutDataType=sfix(16)  OutScaling=2^0
  Psv : Inport  Port=5  OutDataType=sfix(16)  OutScaling=2^0
  Pev : Inport  Port=6  OutDataType=sfix(16)  OutScaling=2^0
  Add : Sum  Inputs=+++++-  OutDataType=sfix(16)  OutScaling=2^-10
  Constant : Constant  OutDataType=sfix(16)  OutScaling=2^0
  Cra : Constant  OutDataType=sfix(16)  OutScaling=2^0
  Divide{,1..5} (6 alike) : Product  Inputs=*/  OutDataType=sfix(16)  OutScaling=2^-10
  Integrator : Integrator
  Product : Product  OutDataType=sfix(16)  OutScaling=2^0  RndMeth=Zero
  Rbv : Constant  Value=0.075  OutDataType=sfix(16)  OutScaling=2^0
  Rev : Constant  Value=0.04  OutDataType=sfix(16)  OutScaling=2^0
  Rhv : Constant  Value=0.224  OutDataType=sfix(16)  OutScaling=2^0
  Rmv : Constant  Value=0.05  OutDataType=sfix(16)  OutScaling=2^0
  Rsv : Constant  Value=0.038  OutDataType=sfix(16)  OutScaling=2^0
  Subtract{,1..4} (5 alike) : Sum  Inputs=+-  OutDataType=sfix(16)  OutScaling=2^-10
  Pra : Outport  OutDataType=sfix(16)  OutScaling=2^0
  wires:
  Divide5/1 -> Add/5
  Rev/1 -> Divide5/2
  Subtract4/1 -> Divide5/1
  Pev/1 -> Subtract4/1
  Divide4/1 -> Add/4
  Rsv/1 -> Divide4/2
  Subtract3/1 -> Divide4/1
  Psv/1 -> Subtract3/1
  Divide3/1 -> Add/3
  Rmv/1 -> Divide3/2
  Subtract2/1 -> Divide3/1
  Pmv/1 -> Subtract2/1
  Divide2/1 -> Add/2
  Rbv/1 -> Divide2/2
  Subtract1/1 -> Divide2/1
  Pbv/1 -> Subtract1/1
  Fi,r/1 -> Add/6
  Add/1 -> Product/2
  Divide1/1 -> Add/1
  Rhv/1 -> Divide1/2
  Subtract/1 -> Divide1/1
  Phv/1 -> Subtract/1
  Divide/1 -> Product/1
  Product/1 -> Integrator/1
  Cra/1 -> Divide/2
  Constant/1 -> Divide/1
  Integrator/1 -> Subtract4/2, Subtract3/2, Subtract2/2, Subtract1/2, Subtract/2, Pra/1

== system cardio/A1_21 ==
  Pra : Inport  OutDataType=sfix(16)  OutScaling=2^0
  Prv : Inport  Port=2  OutDataType=sfix(16)  OutScaling=2^0
  Constant : Constant  Value=0  OutDataType=sfix(16)  OutScaling=2^0
  Divide : Product  Inputs=*/  OutDataType=sfix(16)  OutScaling=2^-10
  Rra : Constant  Value=0.0025  OutDataType=sfix(16)  OutScaling=2^0
  Subtract : Sum  Inputs=+-  OutDataType=sfix(16)  OutScaling=2^-10
  Switch : Switch  OutDataType=sfix(16)  OutScaling=2^0
  Fi,r : Outport  OutDataType=sfix(16)  OutScaling=2^0
  wires:
  Constant/1 -> Switch/3
  Divide/1 -> Switch/1
  Switch/1 -> Fi,r/1
  Rra/1 -> Divide/2
  Subtract/1 -> Divide/1, Switch/2
  Prv/1 -> Subtract/2
  Pra/1 -> Subtract/1

== system cardio/A1_22 ==
  Fi,r : Inport  OutDataType=sfix(16)  OutScaling=2^0
  Fo,r : Inport  Port=2  OutDataType=sfix(16)  OutScaling=2^0
  Integrator : Integrator  InitialCondition=0.1
  Subtract : Sum  Inputs=+-  OutDataType=sfix(16)  OutScaling=2^-10
  Vrv : Outport  OutDataType=sfix(16)  OutScaling=2^0
  wires:
  Integrator/1 -> Vrv/1
  Subtract/1 -> Integrator/1
  Fo,r/1 -> Subtract/2
  Fi,r/1 -> Subtract/1

== system cardio/A1_23 ==
  Pmax,rv : Inport  OutDataType=sfix(16)  OutScaling=2^0
  Ppa : Inport  Port=2  OutDataType=sfix(16)  OutScaling=2^0
  Rrv : Inport  Port=3  OutDataType=sfix(16)  OutScaling=2^0
  Constant : Constant  Value=0  OutDataType=sfix(16)  OutScaling=2^0
  Divide : Product  Inputs=*/  OutDataType=sfix(16)  OutScaling=2^-10
  Subtract : Sum  Inputs=+-  OutDataType=sfix(16)  OutScaling=2^-10
  Switch : Switch  OutDataType=sfix(16)  OutScaling=2^0
  Fo,r : Outport  OutDataType=sfix(16)  OutScaling=2^0
  wires:
  Constant/1 -> Switch/3
  Divide/1 -> Switch/1
  Switch/1 -> Fo,r/1
  Rrv/1 -> Divide/2
  Subtract/1 -> Divide/1, Switch/2
  Ppa/1 -> Subtract/2
  Pmax,rv/1 -> Subtract/1

== system cardio/A1_24 ==
  Pmax,rv : Inport  OutDataType=fixdt(1, 16)  OutScaling=2^0
  Product : Product  OutDataType=fixdt(1, 16)  OutScaling=2^0  RndMeth=Zero
  kR,rv : Constant  Value=0.0014  OutDataType=fixdt(1, 16)  OutScaling=2^0
  Rrv : Outport  OutDataType=fixdt(1, 16)  OutScaling=2^0
  wires:
  kR,rv/1 -> Product/2
  Pmax,rv/1 -> Product/1
  Product/1 -> Rrv/1

== system cardio/A1_25 ==
  fi(t) : Inport  OutDataType=fixdt(1, 16)  OutScaling=2^0
  Vrv : Inport  Port=2  OutDataType=fixdt(1, 16)  OutScaling=2^0
  Emax,rv : Inport  Port=3  OutDataType=fixdt(1, 16)  OutScaling=2^0
  Add : Sum  OutDataType=fixdt(1, 16)  OutScaling=2^-10
  Add1 : Sum  Inputs=+-  OutDataType=fixdt(1, 16)  OutScaling=2^-10
  Constant : Constant  OutDataType=fixdt(1, 16)  OutScaling=2^0
  Constant1 : Constant  OutDataType=fixdt(1, 16)  OutScaling=2^0
  Math Function : Math  OutDataType=fixdt(1, 16)  OutScaling=2^0  SaturateOnIntegerOverflow=on
  Po,rv : Constant  Value=1.5  OutDataType=fixdt(1, 16)  OutScaling=2^0
  Product : Product  Inputs=3  OutDataType=fixdt(1, 16)  OutScaling=2^0  RndMeth=Zero
  Product1 : Product  Inputs=3  OutDataType=fixdt(1, 16)  OutScaling=2^0  RndMeth=Zero
  Product2 : Product  OutDataType=fixdt(1, 16)  OutScaling=2^0  RndMeth=Zero
  Subtract : Sum  Inputs=+-  OutDataType=fixdt(1, 16)  OutScaling=2^-10
  Subtract1 : Sum  Inputs=+-  OutDataType=fixdt(1, 16)  OutScaling=2^-10
  Vu,rv : Constant  Value=40.8  OutDataType=fixdt(1, 16)  OutScaling=2^0
  kE,rv : Constant  Value=0.011  OutDataType=fixdt(1, 16)  OutScaling=2^0
  Pmax,rv : Outport  OutDataType=fixdt(1, 16)  OutScaling=2^0
  wires:
  Math Function/1 -> Add1/1
  Product2/1 -> Math Function/1
  kE,rv/1 -> Product2/2
  Constant1/1 -> Add1/2
  Add1/1 -> Product1/3
  Po,rv/1 -> Product1/2
  Constant/1 -> Subtract1/1
  Subtract1/1 -> Product1/1
  Product1/1 -> Add/2
  Product/1 -> Add/1
  Add/1 -> Pmax,rv/1
  Subtract/1 -> Product/3
  Vu,rv/1 -> Subtract/2
  Vrv/1 -> Product2/1, Subtract/1
  Emax,rv/1 -> Product/2
  fi(t)/1 -> Subtract1/2, Product/1

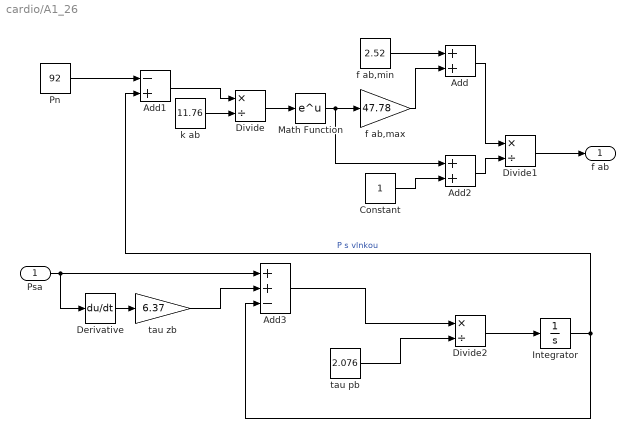
== system cardio/A1_26 ==
  Psa : Inport  OutDataType=sfix(16)  OutScaling=2^0
  Add : Sum  OutDataType=sfix(16)  OutScaling=2^-10
  Add1 : Sum  Inputs=-+  OutDataType=sfix(16)  OutScaling=2^-10
  Add2 : Sum  OutDataType=sfix(16)  OutScaling=2^-10
  Add3 : Sum  Inputs=++-  OutDataType=sfix(16)  OutScaling=2^-10
  Constant : Constant  OutDataType=sfix(16)  OutScaling=2^0
  Derivative : Derivative
  Divide : Product  Inputs=*/  OutDataType=sfix(16)  OutScaling=2^-10
  Divide1 : Product  Inputs=*/  OutDataType=sfix(16)  OutScaling=2^-10
  Divide2 : Product  Inputs=*/  OutDataType=sfix(16)  OutScaling=2^-10
  Integrator : Integrator
  Math Function : Math  OutDataType=sfix(16)  OutScaling=2^0  SaturateOnIntegerOverflow=on
  Pn : Constant  Value=92  OutDataType=sfix(16)  OutScaling=2^0
  f ab,max : Gain  Gain=47.78  ParameterDataType=sfix(16)  ParameterScaling=2^0  OutDataType=sfix(16)  OutScaling=2^0
  f ab,min : Constant  Value=2.52  OutDataType=sfix(16)  OutScaling=2^0
  k ab : Constant  Value=11.76  OutDataType=sfix(16)  OutScaling=2^0
  tau pb : Constant  Value=2.076  OutDataType=sfix(16)  OutScaling=2^0
  tau zb : Gain  Gain=6.37  ParameterDataType=sfix(16)  ParameterScaling=2^0  OutDataType=sfix(16)  OutScaling=2^0
  f ab : Outport  OutDataType=sfix(16)  OutScaling=2^0
  wires:
  Integrator/1 -> Add1/2, Add3/3  "P s vlnkou"
  Divide2/1 -> Integrator/1
  Add3/1 -> Divide2/1
  tau zb/1 -> Add3/2
  Derivative/1 -> tau zb/1
  Psa/1 -> Derivative/1, Add3/1
  tau pb/1 -> Divide2/2
  Constant/1 -> Add2/2
  Add2/1 -> Divide1/2
  Divide1/1 -> f ab/1
  Add/1 -> Divide1/1
  Pn/1 -> Add1/1
  Add1/1 -> Divide/1
  k ab/1 -> Divide/2
  Divide/1 -> Math Function/1
  Math Function/1 -> Add2/1, f ab,max/1
  f ab,max/1 -> Add/2
  f ab,min/1 -> Add/1

== system cardio/A_27 ==
  note: fi ac
  1 : Constant  OutDataType=sfix(16)  OutScaling=2^0
  1/tau c : Gain  Gain=1/2  ParameterDataType=sfix(16)  ParameterScaling=2^0  OutDataType=sfix(16)  OutScaling=2^0
  Add : Sum  Inputs=-+  OutDataType=sfix(16)  OutScaling=2^-10
  Add1 : Sum  OutDataType=sfix(16)  OutScaling=2^-10
  Add2 : Sum  OutDataType=sfix(16)  OutScaling=2^-10
  Add3 : Sum  Inputs=+-  OutDataType=sfix(16)  OutScaling=2^-10
  Divide : Product  Inputs=*/  OutDataType=sfix(16)  OutScaling=2^-10
  Divide1 : Product  Inputs=*/  OutDataType=sfix(16)  OutScaling=2^-10
  Math Function : Math  OutDataType=sfix(16)  OutScaling=2^0  SaturateOnIntegerOverflow=on
  P as O2 : Constant  Value=110  OutDataType=sfix(16)  OutScaling=2^0
  P as O2n : Constant  Value=45  OutDataType=sfix(16)  OutScaling=2^0
  f ac,max : Constant  Value=17.07  OutDataType=sfix(16)  OutScaling=2^0
  f ac,min : Gain  Gain=1.16  ParameterDataType=sfix(16)  ParameterScaling=2^0  OutDataType=sfix(16)  OutScaling=2^0
  f ac1 : Integrator
  k ac : Constant  Value=29.27  OutDataType=sfix(16)  OutScaling=2^0
  f ac : Outport  OutDataType=sfix(16)  OutScaling=2^0
  wires:
  Divide/1 -> Add/2
  P as O2n/1 -> Add3/2
  P as O2/1 -> Add3/1
  Add3/1 -> Divide1/1
  k ac/1 -> Divide1/2
  Divide1/1 -> Math Function/1
  1/1 -> Add2/2
  Add2/1 -> Divide/2
  Add1/1 -> Divide/1
  f ac,min/1 -> Add1/2
  f ac,max/1 -> Add1/1
  Math Function/1 -> Add2/1, f ac,min/1
  1/tau c/1 -> f ac1/1
  Add/1 -> 1/tau c/1
  f ac1/1 -> Add/1, f ac/1

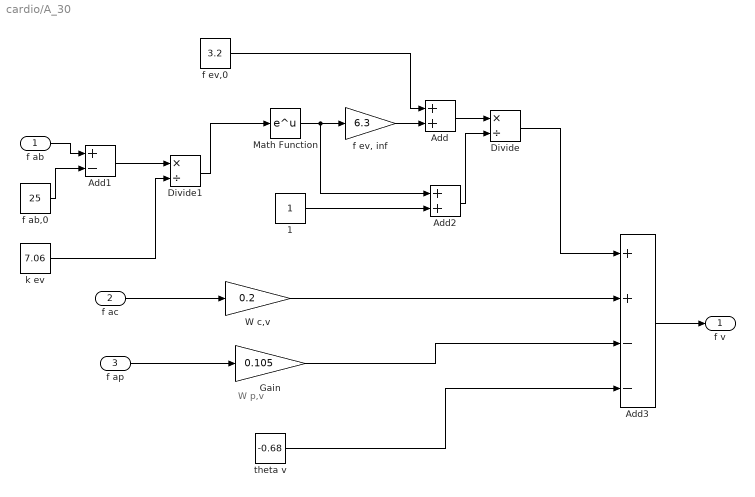
== system cardio/A_30 ==
  note: W p,v
  f ab : Inport  OutDataType=sfix(16)  OutScaling=2^0
  f ac : Inport  Port=2  OutDataType=sfix(16)  OutScaling=2^0
  f ap : Inport  Port=3  OutDataType=sfix(16)  OutScaling=2^0
  1 : Constant  OutDataType=sfix(16)  OutScaling=2^0
  Add : Sum  OutDataType=sfix(16)  OutScaling=2^-10
  Add1 : Sum  Inputs=+-  OutDataType=sfix(16)  OutScaling=2^-10
  Add2 : Sum  OutDataType=sfix(16)  OutScaling=2^-10
  Add3 : Sum  Inputs=++--  OutDataType=sfix(16)  OutScaling=2^-10
  Divide : Product  Inputs=*/  OutDataType=sfix(16)  OutScaling=2^-10
  Divide1 : Product  Inputs=*/  OutDataType=sfix(16)  OutScaling=2^-10
  Gain : Gain  Gain=0.105  ParameterDataType=sfix(16)  ParameterScaling=2^0  OutDataType=sfix(16)  OutScaling=2^0
  Math Function : Math  OutDataType=sfix(16)  OutScaling=2^0  SaturateOnIntegerOverflow=on
  W c,v : Gain  Gain=0.2  ParameterDataType=sfix(16)  ParameterScaling=2^0  OutDataType=sfix(16)  OutScaling=2^0
  f ab,0 : Constant  Value=25  OutDataType=sfix(16)  OutScaling=2^0
  "f ev, inf" : Gain  Gain=6.3  ParameterDataType=sfix(16)  ParameterScaling=2^0  OutDataType=sfix(16)  OutScaling=2^0
  f ev,0 : Constant  Value=3.2  OutDataType=sfix(16)  OutScaling=2^0
  k ev : Constant  Value=7.06  OutDataType=sfix(16)  OutScaling=2^0
  theta v : Constant  Value=-0.68  OutDataType=sfix(16)  OutScaling=2^0
  f v : Outport  OutDataType=sfix(16)  OutScaling=2^0
  wires:
  theta v/1 -> Add3/4
  Gain/1 -> Add3/3
  f ap/1 -> Gain/1
  f ac/1 -> W c,v/1
  W c,v/1 -> Add3/2
  Add3/1 -> f v/1
  Divide/1 -> Add3/1
  1/1 -> Add2/2
  Add2/1 -> Divide/2
  k ev/1 -> Divide1/2
  Divide1/1 -> Math Function/1
  Add1/1 -> Divide1/1
  f ab,0/1 -> Add1/2
  f ab/1 -> Add1/1
  Math Function/1 -> Add2/1, "f ev, inf"/1
  "f ev, inf"/1 -> Add/2
  f ev,0/1 -> Add/1
  Add/1 -> Divide/1
